simulink model "untitled"  (R2022b)
settings: Solver=ode45  StartTime=0.0  StopTime=4  FixedStep=0.02  MaxStep=0.002  RelTol=1e-6
InitFcn:
  | m = 0.5;
  | f = 10;
  | k = 10000;
  | g = 9.81;
  | R = 0.1;
  | H0 = 1;
StartFcn:
  | for i=y(:,2)'
  |     rysuj(i,R,H0)
  | end
settings Model: Creator=local  LastModifiedBy=local
settings DataIOCC: ReturnWorkspaceOutputs=off

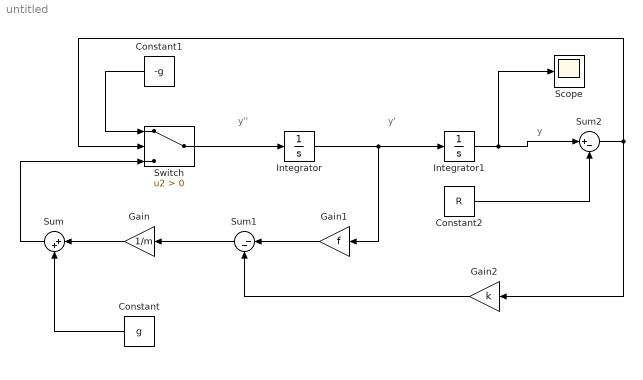
== system untitled ==
  note: y
  note: y'
  note: y''
  Constant : Constant  Value=g
  Constant1 : Constant  Value=-g
  Constant2 : Constant  Value=R
  Gain : Gain  Gain=1/m
  Gain1 : Gain  Gain=f
  Gain2 : Gain  Gain=k
  Integrator : Integrator
  Integrator1 : Integrator  InitialCondition=H0
  Scope : Scope
  Sum : Sum  Inputs=|++
  Sum1 : Sum  Inputs=|--
  Sum2 : Sum  Inputs=|+-
  Switch : Switch  Criteria=u2 > Threshold  SaturateOnIntegerOverflow=off  InputSameDT=off
  wires:
  Switch/1 -> Integrator/1
  Constant1/1 -> Switch/1
  Integrator/1 -> Gain1/1, Integrator1/1
  Integrator1/1 -> Scope/1, Sum2/1
  Constant2/1 -> Sum2/2
  Sum2/1 -> Gain2/1, Switch/2
  Gain1/1 -> Sum1/1
  Gain2/1 -> Sum1/2
  Sum1/1 -> Gain/1
  Gain/1 -> Sum/1
  Constant/1 -> Sum/2
  Sum/1 -> Switch/3
